simulink library "SimMainLibrary"  (R2017b)
settings: Solver=ode45  StartTime=0.0  StopTime=10.0  RelTol=1e-3  EnableMultiTasking=on
values from neighbouring files (symbols this model uses):
  A = eye(16,16)    [full_input_list.m]
  B = zeros(16,1)    [full_input_list.m]
  C = blkdiag(eye(3,3),zeros(3,3),eye(10,10))    [full_input_list.m]
  centerMass = 2.7719    [full_input_list.m]
  H = C    [full_input_list.m]
  homeClock = clock    [full_input_list.m]    (also in initSimulink.m)
  kane_density = 1000    [full_input_list.m]
  m = 4*1/6    (= 0.666666666667)    [initACS.m]
  mewE = 3.986004418e14    (= 398600441800000)    [full_input_list.m]    (also in initACS.m)
  Q_k = zeros(16,16)    [full_input_list.m]
  R = R_k    [full_input_list.m]
  side1Dim = [ 10 10 6.124 ]/100    [full_input_list.m]
  side1Mass = 0.3283    [full_input_list.m]
  side2Dim = [ 10 10 6.124 ]/100    [full_input_list.m]
  st = 1/freq    (= 0.0125)    [full_input_list.m]    (also in initSimulink.m)
  state1_i = [ 0 0 0 , 0 0 0 , q4_0', w0_N]'    [full_input_list.m]
  state2_i = [ 0 0 (teth_length+side1Dim(1)/2+centerDim(3)/2+10*eps) , 0 -.1 0 ,      q4_0_Cube2' , w0_N ]'    [full_input_list.m]
  state3_i = [ 0 0 -(teth_length+side1Dim(1)/2+centerDim(3)/2+10*eps), 0 .1 0 ,      q4_0_Cube3' , w0_N ]'    [full_input_list.m]
  teth_length = 1    [full_input_list.m]
  teth_numLinks = 3    [full_input_list.m]
  u_k = zeros(16,1)    [full_input_list.m]
  w_k = zeros(16,1)    [full_input_list.m]
  Z_k = zeros(16,1)    [full_input_list.m]
undefined symbols (not defined in the file or in its folder): DiscIntNeverNeededParam, IAU, spring1kd, spring1ks, X, Y, Z
libraries: sm_lib x113, SimMainLibrary x27, nesl_utility x24, simulink x9, sharedutil x2, dspmtrx3 x1, dspinverses x1, aerolibtransform2 x1, aerolibgravity2 x1
(part 7 of 7)

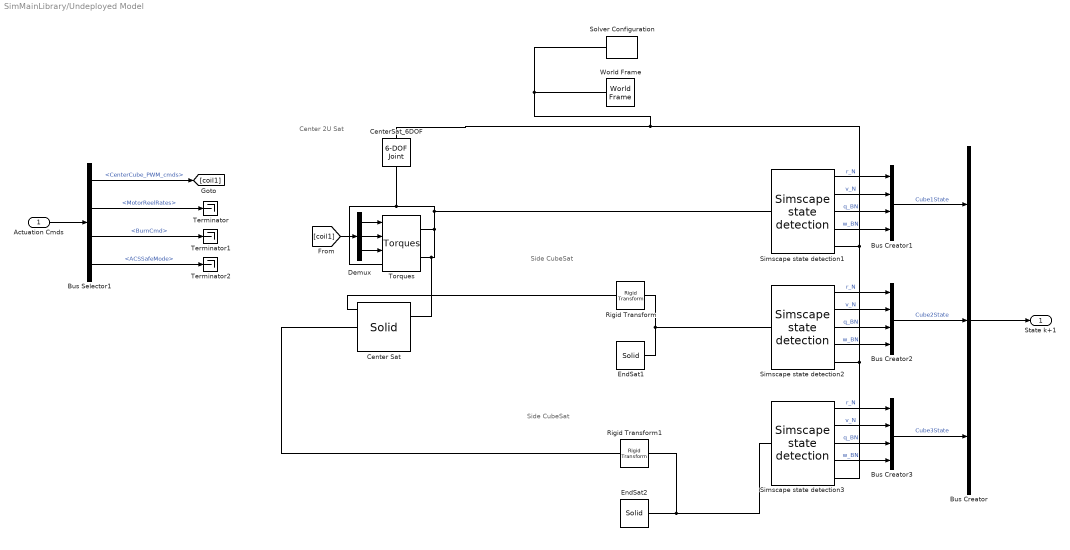
== system SimMainLibrary/Undeployed Model ==
  note: Side CubeSat
  note: Side CubeSat
  note: Center 2U Sat
  Actuation Cmds : Inport
  Bus Creator : BusCreator  Inputs=3
  Bus Creator1 : BusCreator  Inputs=4
  Bus Creator2 : BusCreator  Inputs=4
  Bus Creator3 : BusCreator  Inputs=4
  Bus Selector1 : BusSelector  OutputSignals=CenterCube_PWM_cmds,MotorReelRates,BurnCmd,ACSSafeMode
  Center Sat : sm_lib/Body Elements/Solid  InertiaType=CalculateFromGeometry  Mass=centerMass  MassUnits=kg  CenterOfMass=[0 0 0]  CenterOfMassUnits=m  MomentsOfInertia=[1 1 1]  MomentsOfInertiaUnits=kg*m^2  ProductsOfInertia=[0 0 0]  ProductsOfInertiaUnits=kg*m^2  DensityBased=off  Density=1000  DensityUnits=kg/(m^3)  DoExposeReferenceFrame=on  SerializedFrames=<Frames><Frame><Id>Frame1</Id><Value><Name>PosZ</Name><Origin><Source>GeometricFeature</Source><FeatureName>+z surface</FeatureName></Origin><PrimaryAxis><DefinedDirection>+Z</DefinedDirection><Source>ReferenceFrame</Source><SourceDirection>+Z</SourceDirection><FeatureName></FeatureName></PrimaryAxis><SecondaryAxis><DefinedDirection>+X</DefinedDirection><Source>ReferenceFrame</Source><SourceDirection>+X</SourceDirection><FeatureName></FeatureName></SecondaryAxis></Value></Frame><Frame><Id>Frame2</Id><Value><Name>NegZ</Name><Origin><Source>GeometricFeature</Source><FeatureName>-z surface</FeatureName></Origin><PrimaryAxis><DefinedDirection>+Z</DefinedDirection><Source>ReferenceFrame</Source><SourceDirection>+Z</SourceDirection><FeatureName></FeatureName></PrimaryAxis><SecondaryAxis><DefinedDirection>+X</DefinedDirection><Source>ReferenceFrame</Source><SourceDirection>+X</SourceDirection><FeatureName></FeatureName></SecondaryAxis></Value></Frame><Frame><Id>Frame3</Id><Value><Name>PosY</Name><Origin><Source>ReferenceFrame</Source><FeatureName></FeatureName></Origin><PrimaryAxis><DefinedDirection>+Z</DefinedDirection><Source>ReferenceFrame</Source><SourceDirection>+Z</SourceDirection><FeatureName></FeatureName></PrimaryAxis><SecondaryAxis><DefinedDirection>+X</DefinedDirection><Source>ReferenceFrame</Source><SourceDirection>+X</SourceDirection><FeatureName></FeatureName></SecondaryAxis></Value></Frame><Frame><Id>Frame4</Id><Value><Name>NegY</Name><Origin><Source>ReferenceFrame</Source><FeatureName></FeatureName></Origin><PrimaryAxis><DefinedDirection>+Z</DefinedDirection><Source>ReferenceFrame</Source><SourceDirection>+Z</SourceDirection><FeatureName></FeatureName></PrimaryAxis><SecondaryAxis><DefinedDirection>+X</DefinedDirection><Source>ReferenceFrame</Source><SourceDirection>+X</SourceDirection><FeatureName></FeatureName></SecondaryAxis></Value></Frame></Frames>  GraphicType=FromGeometry  MarkerShape=Sphere  MarkerSize=10  GraphicVisPropType=SimpleVisualProperties  GraphicDiffuseColor=[0.5 0.5 0.5]  GraphicSpecularColor=[0.5 0.5 0.5 1.0]  GraphicAmbientColor=[0.15 0.15 0.15 1.0]  GraphicEmissiveColor=[0.0 0.0 0.0 1.0]  GraphicShininess=75  GraphicOpacity=1.0  GeometryShape=Brick  RectangleSize=[1 1]  RectangleSizeUnits=m  BrickDimensions=centerDim  BrickDimensionUnits=m  CylinderRadius=1  CylinderRadiusUnits=m  CylinderLength=1  CylinderLengthUnits=m  SphereRadius=1  SphereRadiusUnits=m  EllipsoidRadii=[1 1 1]  EllipsoidRadiiUnits=m  ExtrusionCrossSection=[1 1; -1 1; -1 -1; 1 -1]  ExtrusionCrossSectionUnits=m  ExtrusionLength=1  ExtrusionLengthUnits=m  PolygonNumSides=3  PolygonOuterRadius=1  PolygonOuterRadiusUnits=m  ExtGeomFileType=STEP  ExtGeomFileUnits=m  RevolutionCrossSection=[1 1; 1 -1; 2 -1; 2 1]  RevolutionCrossSectionUnits=m  RevolutionExtent=Full  RevolutionAngle=180  RevolutionAngleUnits=deg
  CenterSat_6DOF : sm_lib/Joints/6-DOF Joint  SenseConstraintForce=off  SenseConstraintForceX=off  SenseConstraintForceY=off  SenseConstraintForceZ=off  SenseConstraintTorque=off  SenseConstraintTorqueX=off  SenseConstraintTorqueY=off  SenseConstraintTorqueZ=off  SenseTotalForce=off  SenseTotalForceX=off  SenseTotalForceY=off  SenseTotalForceZ=off  SenseTotalTorque=off  SenseTotalTorqueX=off  SenseTotalTorqueY=off  SenseTotalTorqueZ=off  CompositeWrenchDir=FollowerOnBase  CompositeWrenchFrame=BaseFrame  PxEquilibriumPosition=0  PxEquilibriumPositionUnits=m  PxSpringStiffness=0  PxSpringStiffnessUnits=N/m  PxDampingCoefficient=0  PxDampingCoefficientUnits=N/(m/s)  PxTorqueActuationMode=NoTorque  PxMotionActuationMode=ComputedMotion  PxSensePosition=off  PxSenseVelocity=off  PxSenseAcceleration=off  PxSenseTorqueForce=off  PxPositionTargetSpecify=on  PxPositionTargetPriority=High  PxPositionTargetValue=state1_i(1)  PxPositionTargetValueUnits=m  PxVelocityTargetSpecify=on  PxVelocityTargetPriority=High  PxVelocityTargetValue=state1_i(4)  PxVelocityTargetValueUnits=m/s  PyEquilibriumPosition=0  PyEquilibriumPositionUnits=m  PySpringStiffness=0  PySpringStiffnessUnits=N/m  PyDampingCoefficient=0  PyDampingCoefficientUnits=N/(m/s)  PyTorqueActuationMode=NoTorque  PyMotionActuationMode=ComputedMotion  PySensePosition=off  PySenseVelocity=off  PySenseAcceleration=off  PySenseTorqueForce=off  PyPositionTargetSpecify=on  PyPositionTargetPriority=High  PyPositionTargetValue=state1_i(2)  PyPositionTargetValueUnits=m  PyVelocityTargetSpecify=on  PyVelocityTargetPriority=High  PyVelocityTargetValue=state1_i(5)  PyVelocityTargetValueUnits=m/s  PzEquilibriumPosition=0  PzEquilibriumPositionUnits=m  PzSpringStiffness=0  PzSpringStiffnessUnits=N/m  PzDampingCoefficient=0  PzDampingCoefficientUnits=N/(m/s)  PzTorqueActuationMode=NoTorque  PzMotionActuationMode=ComputedMotion  PzSensePosition=off  PzSenseVelocity=off  PzSenseAcceleration=off  PzSenseTorqueForce=off  PzPositionTargetSpecify=on  PzPositionTargetPriority=High  PzPositionTargetValue=state1_i(3)  PzPositionTargetValueUnits=m  PzVelocityTargetSpecify=on  PzVelocityTargetPriority=High  PzVelocityTargetValue=state1_i(6)  PzVelocityTargetValueUnits=m/s  SphDefPosRotationMethod=None  SphDefPosRotationAngleUnits=deg  SphDefPosRotationStandardAxis=+Z  SphDefPosRotationAngle=0.0  SphDefPosRotationArbitraryAxis=[0 0 1]  SphDefPosFollAlignAxisA=+X  SphDefPosBaseAlignAxisA=+Y  SphDefPosFollAlignAxisB=+Y  SphDefPosBaseAlignAxisB=+Z  SphDefPosRotationSequenceAxes=FollowerAxes  SphDefPosRotationSequence=XYX  SphDefPosRotationSequenceAngles=[0 0 0]  SphDefPosRotationSequenceAnglesUnits=deg  SphDefPosRotationMatrix=[1 0 0; 0 1 0; 0 0 1]  SphEqPosRotationMethod=None  SphEqPosRotationAngleUnits=deg  SphEqPosRotationStandardAxis=+Z  SphEqPosRotationAngle=0.0  SphEqPosRotationArbitraryAxis=[0 0 1]  SphEqPosFollAlignAxisA=+X  SphEqPosBaseAlignAxisA=+Y  SphEqPosFollAlignAxisB=+Y  SphEqPosBaseAlignAxisB=+Z  SphEqPosRotationSequenceAxes=FollowerAxes  SphEqPosRotationSequence=XYX  SphEqPosRotationSequenceAngles=[0 0 0]  SphEqPosRotationSequenceAnglesUnits=deg  SphEqPosRotationMatrix=[1 0 0; 0 1 0; 0 0 1]  SphSpringStiffness=0  SphSpringStiffnessUnits=N*m/deg  SphDampingCoefficient=0  SphDampingCoefficientUnits=N*m/(deg/s)  SphActuateTorqueX=off  SphActuateTorqueY=off  SphActuateTorqueZ=off  SphActuateTorque=off  SphTorqueActuationMode=NoTorque  SphMotionActuationMode=ComputedMotion  SphActuationFrame=BaseFrame  SphSensePosition=off  SphSenseVelocityX=off  SphSenseVelocityY=off  SphSenseVelocityZ=off  SphSenseVelocity=off  SphSenseAccelerationX=off  SphSenseAccelerationY=off  SphSenseAccelerationZ=off  SphSenseAcceleration=off  SphSenseTorqueX=off  SphSenseTorqueY=off  SphSenseTorqueZ=off  SphSenseTorqueForce=off  SphSensingFrame=BaseFrame  SphPositionTargetRotationMethod=RotationMatrix  SphPositionTargetRotationAngleUnits=deg  SphPositionTargetRotationStandardAxis=+Z  SphPositionTargetRotationAngle=0.0  SphPositionTargetRotationArbitraryAxis=[0 0 1]  SphPositionTargetFollAlignAxisA=+X  SphPositionTargetBaseAlignAxisA=+Y  SphPositionTargetFollAlignAxisB=+Y  SphPositionTargetBaseAlignAxisB=+Z  SphPositionTargetRotationSequenceAxes=FollowerAxes  SphPositionTargetRotationSequence=XYX  SphPositionTargetRotationSequenceAngles=[0 0 0]  SphPositionTargetRotationSequenceAnglesUnits=deg  SphPositionTargetRotationMatrix=state1_i_rotation  SphPositionTargetSpecify=on  SphPositionTargetPriority=High  SphVelocityTargetValue=state1_i(11:13)  SphVelocityTargetValueUnits=rad/s  SphVelocityTargetSpecify=on  SphVelocityTargetPriority=High  SphVelocityTargetInFollowerFrame=on
  Demux : Demux  Outputs=3
  EndSat1 : sm_lib/Body Elements/Solid  InertiaType=CalculateFromGeometry  Mass=side1Mass  MassUnits=kg  CenterOfMass=[0 0 0]  CenterOfMassUnits=m  MomentsOfInertia=[1 1 1]  MomentsOfInertiaUnits=kg*m^2  ProductsOfInertia=[0 0 0]  ProductsOfInertiaUnits=kg*m^2  DensityBased=off  Density=1000  DensityUnits=kg/(m^3)  DoExposeReferenceFrame=on  SerializedFrames=<Frames><Frame><Id>Frame1</Id><Value><Name>F1</Name><Origin><Source>GeometricFeature</Source><FeatureName>-y surface</FeatureName></Origin><PrimaryAxis><DefinedDirection>+Z</DefinedDirection><Source>ReferenceFrame</Source><SourceDirection>-Z</SourceDirection><FeatureName></FeatureName></PrimaryAxis><SecondaryAxis><DefinedDirection>+X</DefinedDirection><Source>ReferenceFrame</Source><SourceDirection>+X</SourceDirection><FeatureName></FeatureName></SecondaryAxis></Value></Frame></Frames>  GraphicType=FromGeometry  MarkerShape=Sphere  MarkerSize=10  GraphicVisPropType=SimpleVisualProperties  GraphicDiffuseColor=[0.5 0.5 0.5]  GraphicSpecularColor=[0.5 0.5 0.5 1.0]  GraphicAmbientColor=[0.15 0.15 0.15 1.0]  GraphicEmissiveColor=[0.0 0.0 0.0 1.0]  GraphicShininess=75  GraphicOpacity=1.0  GeometryShape=Brick  RectangleSize=[1 1]  RectangleSizeUnits=m  BrickDimensions=side1Dim  BrickDimensionUnits=m  CylinderRadius=1  CylinderRadiusUnits=m  CylinderLength=1  CylinderLengthUnits=m  SphereRadius=1  SphereRadiusUnits=m  EllipsoidRadii=[1 1 1]  EllipsoidRadiiUnits=m  ExtrusionCrossSection=[1 1; -1 1; -1 -1; 1 -1]  ExtrusionCrossSectionUnits=m  ExtrusionLength=1  ExtrusionLengthUnits=m  PolygonNumSides=3  PolygonOuterRadius=1  PolygonOuterRadiusUnits=m  ExtGeomFileType=STEP  ExtGeomFileUnits=m  RevolutionCrossSection=[1 1; 1 -1; 2 -1; 2 1]  RevolutionCrossSectionUnits=m  RevolutionExtent=Full  RevolutionAngle=180  RevolutionAngleUnits=deg
  EndSat2 : sm_lib/Body Elements/Solid  InertiaType=CalculateFromGeometry  Mass=side1Mass  MassUnits=kg  CenterOfMass=[0 0 0]  CenterOfMassUnits=m  MomentsOfInertia=[1 1 1]  MomentsOfInertiaUnits=kg*m^2  ProductsOfInertia=[0 0 0]  ProductsOfInertiaUnits=kg*m^2  DensityBased=off  Density=1000  DensityUnits=kg/(m^3)  DoExposeReferenceFrame=on  SerializedFrames=<Frames><Frame><Id>Frame1</Id><Value><Name>F1</Name><Origin><Source>GeometricFeature</Source><FeatureName>-y surface</FeatureName></Origin><PrimaryAxis><DefinedDirection>+Z</DefinedDirection><Source>ReferenceFrame</Source><SourceDirection>-Z</SourceDirection><FeatureName></FeatureName></PrimaryAxis><SecondaryAxis><DefinedDirection>+X</DefinedDirection><Source>ReferenceFrame</Source><SourceDirection>+X</SourceDirection><FeatureName></FeatureName></SecondaryAxis></Value></Frame></Frames>  GraphicType=FromGeometry  MarkerShape=Sphere  MarkerSize=10  GraphicVisPropType=SimpleVisualProperties  GraphicDiffuseColor=[0.5 0.5 0.5]  GraphicSpecularColor=[0.5 0.5 0.5 1.0]  GraphicAmbientColor=[0.15 0.15 0.15 1.0]  GraphicEmissiveColor=[0.0 0.0 0.0 1.0]  GraphicShininess=75  GraphicOpacity=1.0  GeometryShape=Brick  RectangleSize=[1 1]  RectangleSizeUnits=m  BrickDimensions=side1Dim  BrickDimensionUnits=m  CylinderRadius=1  CylinderRadiusUnits=m  CylinderLength=1  CylinderLengthUnits=m  SphereRadius=1  SphereRadiusUnits=m  EllipsoidRadii=[1 1 1]  EllipsoidRadiiUnits=m  ExtrusionCrossSection=[1 1; -1 1; -1 -1; 1 -1]  ExtrusionCrossSectionUnits=m  ExtrusionLength=1  ExtrusionLengthUnits=m  PolygonNumSides=3  PolygonOuterRadius=1  PolygonOuterRadiusUnits=m  ExtGeomFileType=STEP  ExtGeomFileUnits=m  RevolutionCrossSection=[1 1; 1 -1; 2 -1; 2 1]  RevolutionCrossSectionUnits=m  RevolutionExtent=Full  RevolutionAngle=180  RevolutionAngleUnits=deg
  Rigid Transform : sm_lib/Frames and Transforms/Rigid Transform  TranslationMethod=Cartesian  TranslationStandardOffset=0  TranslationLengthUnit=m  TranslationStandardAxis=+Z  TranslationCartesianOffset=[0 0 side1Dim(3)/2]  TranslationROffset=0  TranslationROffsetUnits=m  TranslationZOffset=0  TranslationZOffsetUnits=m  TranslationThetaOffset=0  TranslationThetaOffsetUnits=deg  RotationMethod=None  RotationAngleUnits=deg  RotationStandardAxis=+Z  RotationAngle=0.0  RotationArbitraryAxis=[0 0 1]  FollAlignAxisA=+X  BaseAlignAxisA=+Y  FollAlignAxisB=+Y  BaseAlignAxisB=+Z  RotationSequenceAxes=FollowerAxes  RotationSequence=XYX  RotationSequenceAngles=[0 0 0]  RotationSequenceAnglesUnits=deg  RotationMatrix=[1 0 0; 0 1 0; 0 0 1]
  Rigid Transform1 : sm_lib/Frames and Transforms/Rigid Transform  TranslationMethod=Cartesian  TranslationStandardOffset=0  TranslationLengthUnit=m  TranslationStandardAxis=+Z  TranslationCartesianOffset=[0 0 -side2Dim(3)/2]  TranslationROffset=0  TranslationROffsetUnits=m  TranslationZOffset=0  TranslationZOffsetUnits=m  TranslationThetaOffset=0  TranslationThetaOffsetUnits=deg  RotationMethod=None  RotationAngleUnits=deg  RotationStandardAxis=+Z  RotationAngle=0.0  RotationArbitraryAxis=[0 0 1]  FollAlignAxisA=+X  BaseAlignAxisA=+Y  FollAlignAxisB=+Y  BaseAlignAxisB=+Z  RotationSequenceAxes=FollowerAxes  RotationSequence=XYX  RotationSequenceAngles=[0 0 0]  RotationSequenceAnglesUnits=deg  RotationMatrix=[1 0 0; 0 1 0; 0 0 1]
  Simscape state detection1 : SimMainLibrary/Simscape state detection
      settings: SourceProductName=CUGravity Library
  Simscape state detection2 : SimMainLibrary/Simscape state detection
      settings: SourceProductName=CUGravity Library
  Simscape state detection3 : SimMainLibrary/Simscape state detection
      settings: SourceProductName=CUGravity Library
  Solver Configuration : nesl_utility/Solver Configuration  PhysicalDomain=network_engine_domain  SubClassName=solver  LeftPortType=input  RightPortType=generic  Accelerate=off  Tones=[]  Harmonics=[]  SimulateNoise=off  Profile=off  UseLocalSampling=off  EnableSwitchedLinearOptims=on  FrequencyDomain=off  UseCCode=off  RelTol=0.001  AbsTol=1e-06  MinStep=1e-09  ToWorkspace=off  RevertToSquareIcSolve=off  NumHomotopyIterations=100  PhasorMode=off  PhasorModeNumHarmonics=1  DoDC=off  ResidualTolerance=1e-09  UseLocalSolver=off  LocalSolverChoice=NE_BACKWARD_EULER_ADVANCER  LocalSolverSampleTime=st  DoFixedCost=off  MaxNonlinIter=3  MaxModeIter=2  LinearAlgebra=Sparse  DelaysMemoryBudget=1024  AutomaticFiltering=off  FilteringTimeConstant=0.001
  Terminator : Terminator
  Terminator1 : Terminator
  Terminator2 : Terminator
  Torques : SimMainLibrary/Single Link Simscape Model/Torques
      settings: SourceProductName=CUGravity Library
  World Frame : sm_lib/Frames and Transforms/World Frame
  State k+1 : Outport
  wires:
  Actuation Cmds/1 -> Bus Selector1/1
  Simscape state detection3/4 -> Bus Creator3/4  "w_BN"
  Simscape state detection3/3 -> Bus Creator3/3  "q_BN"
  Simscape state detection3/2 -> Bus Creator3/2  "v_N"
  Simscape state detection3/1 -> Bus Creator3/1  "r_N"
  Simscape state detection2/4 -> Bus Creator2/4  "w_BN"
  Simscape state detection2/3 -> Bus Creator2/3  "q_BN"
  Simscape state detection2/2 -> Bus Creator2/2  "v_N"
  Simscape state detection2/1 -> Bus Creator2/1  "r_N"
  Simscape state detection1/4 -> Bus Creator1/4  "w_BN"
  Simscape state detection1/3 -> Bus Creator1/3  "q_BN"
  Simscape state detection1/2 -> Bus Creator1/2  "v_N"
  Simscape state detection1/1 -> Bus Creator1/1  "r_N"
  Bus Creator3/1 -> Bus Creator/3  "Cube3State"
  Bus Creator2/1 -> Bus Creator/2  "Cube2State"
  Bus Creator1/1 -> Bus Creator/1  "Cube1State"
  Bus Creator/1 -> State k+1/1
  Demux/2 -> Torques/2
  Demux/3 -> Torques/3
  Demux/1 -> Torques/1
  [coil1] -> Demux/1
  Bus Selector1/1 -> [coil1]  "<CenterCube_PWM_cmds>"
  Bus Selector1/2 -> Terminator/1  "<MotorReelRates>"
  Bus Selector1/3 -> Terminator1/1  "<BurnCmd>"
  Bus Selector1/4 -> Terminator2/1  "<ACSSafeMode>"
  connections:
  Torques/RConn2 -- Center Sat/RConn1 -- Torques/RConn1 -- CenterSat_6DOF/RConn1 -- Torques/LConn1 -- Simscape state detection1/LConn1
  Solver Configuration/RConn1 -- Simscape state detection3/RConn1 -- Simscape state detection2/RConn1 -- Simscape state detection1/RConn1 -- CenterSat_6DOF/LConn1 -- World Frame/RConn1
  EndSat1/RConn1 -- Rigid Transform/RConn1 -- Simscape state detection2/LConn1
  EndSat2/RConn1 -- Rigid Transform1/RConn1 -- Simscape state detection3/LConn1
  Rigid Transform/LConn1 -- Center Sat/LConn1
  Rigid Transform1/LConn1 -- Center Sat/LConn2

== system SimMainLibrary/Update Tether properties ==
  note: Update Tether properties
  note: Update Tether Properties
      | This block updates the dynamic properties of the tether in response to input from MotorReelRates.
      | It outputs a continuous signal of the current tether length for use in the SimScape models.
      | If there is a non-zero reeling signal, it updates the dynamic variables in the workspace.
  <MotorReelRates> : Inport
  Abs : Abs
  Add : Sum
  Add1 : Sum
  Add2 : Sum
  Constant1 : Constant  Value=teth_length
  Constant4 : Constant  Value=teth_length
  If : If  IfExpression=u1 > 1e-5  ShowElse=off
  If Action Subsystem : Subsystem  TreatAsAtomicUnit=on
  Length Signal Filter : TransferFcn  Denominator=[.02 .25 1]
  Mux : Mux  Inputs=3
  Terminator : Terminator  Commented=on
  Unit Delay : UnitDelay  SampleTime=-1
  Tether length : Outport
  Out1 : Outport  Port=2
  wires:
  If/1 -> If Action Subsystem/Action
  <MotorReelRates>/1 -> Mux/1, Add/2, If Action Subsystem/1(Length Increment), Abs/1  "Controller Signal"
  Constant4/1 -> Add1/1
  Add/1 -> Length Signal Filter/1, Add1/2, Mux/2, Unit Delay/1  "Added Length"
  Add1/1 -> If Action Subsystem/2(Length)  "Length"
  Unit Delay/1 -> Add/1
  Abs/1 -> If/1
  Mux/1 -> Out1/1
  Add2/1 -> Tether length/1, Mux/3
  Length Signal Filter/1 -> Add2/1
  Constant1/1 -> Add2/2

== system SimMainLibrary/cross product matrix ==
  a : Inport
  Constant : Constant  Value=0
  Constant1 : Constant  Value=0
  Constant7 : Constant  Value=0
  Demux : Demux  Outputs=3
  Gain2 : Gain  Gain=-1
  Gain3 : Gain  Gain=-1
  Gain4 : Gain  Gain=-1
  crs : sharedutil/Create 3x3 Matrix
  ax : Outport
  wires:
  crs/1 -> ax/1
  Constant/1 -> crs/1
  Constant1/1 -> crs/5
  Constant7/1 -> crs/9
  Gain2/1 -> crs/2
  Demux/1 -> crs/8, Gain3/1
  Demux/2 -> crs/3, Gain4/1
  Gain4/1 -> crs/7
  a/1 -> Demux/1
  Demux/3 -> crs/4, Gain2/1
  Gain3/1 -> crs/6

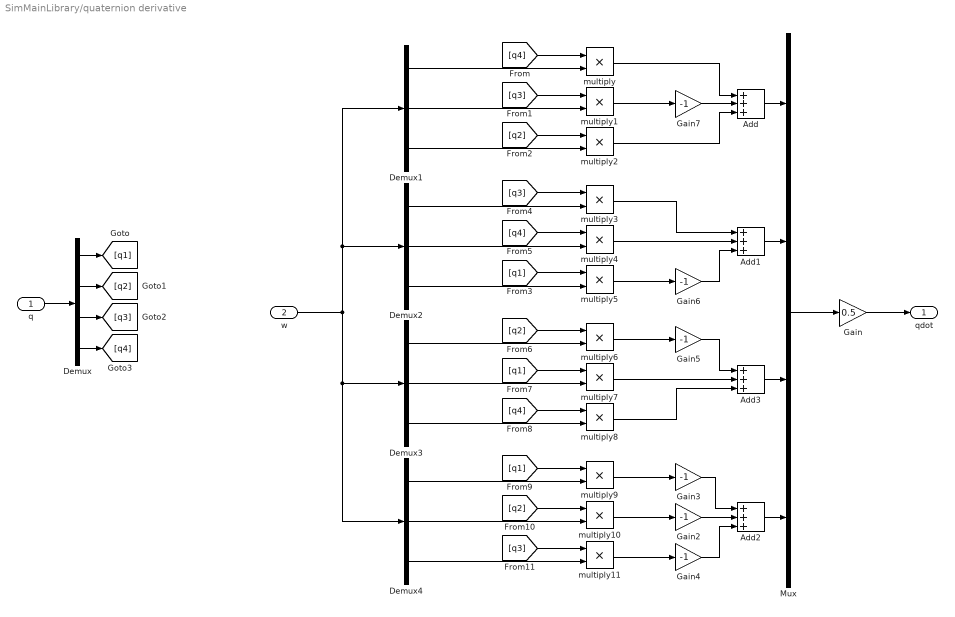
== system SimMainLibrary/quaternion derivative ==
  q : Inport
  w : Inport  Port=2
  Add{,1..3} (4 alike) : Sum  Inputs=+++
  Demux : Demux
  Demux{1..4} (4 alike) : Demux  Outputs=3
  Gain : Gain  Gain=0.5
  Gain{2..7} (6 alike) : Gain  Gain=-1
  Mux : Mux
  multiply{,1..11} (12 alike) : Product  Inputs=**
  qdot : Outport
  wires:
  Add/1 -> Mux/1
  Gain2/1 -> Add2/2
  Gain6/1 -> Add1/3
  Add3/1 -> Mux/3
  Add2/1 -> Mux/4
  Add1/1 -> Mux/2
  multiply/1 -> Add/1
  multiply1/1 -> Gain7/1
  Gain4/1 -> Add2/3
  Gain3/1 -> Add2/1
  Gain7/1 -> Add/2
  Mux/1 -> Gain/1
  multiply4/1 -> Add1/2
  multiply5/1 -> Gain6/1
  Gain5/1 -> Add3/1
  multiply7/1 -> Add3/2
  multiply10/1 -> Gain2/1
  multiply8/1 -> Add3/3
  multiply3/1 -> Add1/1
  multiply2/1 -> Add/3
  multiply9/1 -> Gain3/1
  multiply11/1 -> Gain4/1
  multiply6/1 -> Gain5/1
  q/1 -> Demux/1
  w/1 -> Demux3/1, Demux4/1, Demux2/1, Demux1/1
  Gain/1 -> qdot/1
  Demux1/2 -> multiply1/2
  Demux1/1 -> multiply/2
  Demux1/3 -> multiply2/2
  Demux2/1 -> multiply3/2
  Demux2/2 -> multiply4/2
  Demux2/3 -> multiply5/2
  Demux3/1 -> multiply6/2
  Demux3/2 -> multiply7/2
  Demux3/3 -> multiply8/2
  Demux4/3 -> multiply11/2
  Demux4/2 -> multiply10/2
  Demux4/1 -> multiply9/2
  Demux/1 -> [q1]
  Demux/2 -> [q2]
  Demux/3 -> [q3]
  Demux/4 -> [q4]
  [q4] -> multiply/1
  [q3] -> multiply1/1
  [q2] -> multiply2/1
  [q1] -> multiply5/1
  [q3] -> multiply3/1
  [q4] -> multiply4/1
  [q2] -> multiply6/1
  [q1] -> multiply7/1
  [q4] -> multiply8/1
  [q1] -> multiply9/1
  [q2] -> multiply10/1
  [q3] -> multiply11/1

== system SimMainLibrary/Sequential Motor Controller/Spinning fast1 ==
  In1 : Inport
  Action Port : ActionPort  InitializeStates=reset
  Out1 : Outport
  wires:
  In1/1 -> Out1/1

== system SimMainLibrary/Sequential Motor Controller/Spinning slow1 ==
  Action Port : ActionPort
  Constant : Constant  Value=0
  Out1 : Outport
  wires:
  Constant/1 -> Out1/1

== system SimMainLibrary/SideCubeEstimators/Kalman Gain and Estamated State Computation ==
  P_kp : Inport
  x_kp : Inport  Port=2
  Y : Inport  Port=3
  " LU Inverse" : dspinverses/ LU Inverse
      settings: SourceProductName=DSP System Toolbox
  Add1 : Sum
  Add3 : Sum  Inputs=-+
  H : Constant  Value=H
  H1 : Constant  Value=H
  Math Function : Math  Operator=transpose  SaturateOnIntegerOverflow=on
  Product{,1,3..4,6} (5 alike) : Product  Multiplication=Matrix(*)
  R : Constant  Value=R
  K : Outport
  x_k : Outport  Port=2
  wires:
  Add3/1 -> x_k/1
  P_kp/1 -> Product1/1, Product3/2
  Product6/1 -> Add3/1
  H1/1 -> Product6/1
  Product3/1 -> Product4/1
  Add1/1 -> " LU Inverse"/1
  Product4/1 -> Add1/1
  R/1 -> Add1/2
  Y/1 -> Add3/2
  x_kp/1 -> Product6/2
  Product/1 -> K/1  "Kalman Gain K"
  Math Function/1 -> Product4/2
  Product1/1 -> Product/1
  " LU Inverse"/1 -> Product/2
  H/1 -> Math Function/1, Product1/2, Product3/1

== system SimMainLibrary/SideCubeEstimators/New State Prediction  ==
  P_k-1 : Inport
  x_k-1 : Inport  Port=2
  A : Constant  Value=A
  Add1 : Sum  Inputs=+++
  Add2 : Sum
  B : Constant  Value=B
  Math Function : Math  Operator=transpose  SaturateOnIntegerOverflow=on
  Product{,1..3} (4 alike) : Product  Multiplication=Matrix(*)
  Q_k : Constant  Value=Q_k
  u_k : Constant  Value=u_k
  w_k : Constant  Value=w_k
  P_kp : Outport
  "x_kp  " : Outport  Port=2
  wires:
  Add2/1 -> P_kp/1
  Product3/1 -> Add2/1
  P_k-1/1 -> Product2/2
  Q_k/1 -> Add2/2
  Add1/1 -> "x_kp  "/1
  w_k/1 -> Add1/3
  u_k/1 -> Product1/2
  Product1/1 -> Add1/2
  B/1 -> Product1/1
  A/1 -> Product/1, Product2/1, Math Function/1
  x_k-1/1 -> Product/2
  Product/1 -> Add1/1
  Math Function/1 -> Product3/2
  Product2/1 -> Product3/1

== system SimMainLibrary/SideCubeEstimators/Y computation ==
  In1 : Inport
  Add2 : Sum
  C : Constant  Value=C
  Product2 : Product  Multiplication=Matrix(*)
  "Z_k " : Constant  Value=Z_k
  Y : Outport
  wires:
  Product2/1 -> Add2/1
  C/1 -> Product2/1
  In1/1 -> Product2/2
  "Z_k "/1 -> Add2/2
  Add2/1 -> Y/1

== system SimMainLibrary/SideCubeSensors/Create Mag Vector ==
  q_BN : Inport
  r_N : Inport  Port=2
  Constant : Constant  Value=[1 1 1]
  Terminator : Terminator
  Terminator1 : Terminator
  mag_B : Outport
  wires:
  q_BN/1 -> Terminator/1
  r_N/1 -> Terminator1/1
  Constant/1 -> mag_B/1

== system SimMainLibrary/SideCubeSensors/Create Sun Vector ==
  q_BN : Inport
  r_N : Inport  Port=2
  time : Inport  Port=3
  Constant1 : Constant  Value=[1 1 1]
  Terminator : Terminator
  Terminator1 : Terminator
  Terminator2 : Terminator
  sun_B : Outport
  wires:
  q_BN/1 -> Terminator/1
  r_N/1 -> Terminator1/1
  Constant1/1 -> sun_B/1
  time/1 -> Terminator2/1

== system SimMainLibrary/SideCubeSensors/Frame Convert ==
  a_N : Inport
  q_BN : Inport  Port=2
  Terminator : Terminator
  a_B : Outport
  wires:
  a_N/1 -> a_B/1
  q_BN/1 -> Terminator/1

== system SimMainLibrary/Single Link Simscape Model/Torques ==
  tau_Y : Inport
  tau_X : Inport  Port=2
  tau_Z : Inport  Port=3
  External Force and Torque : sm_lib/Forces and Torques/External Force and Torque  ForceResolutionFrame=AttachedFrame  EnableForceX=off  EnableForceY=off  EnableForceZ=off  EnableForce=off  TorqueResolutionFrame=AttachedFrame  EnableTorqueX=off  EnableTorqueY=on  EnableTorqueZ=off  EnableTorque=off
  External Force and Torque1 : sm_lib/Forces and Torques/External Force and Torque  ForceResolutionFrame=AttachedFrame  EnableForceX=off  EnableForceY=off  EnableForceZ=off  EnableForce=off  TorqueResolutionFrame=AttachedFrame  EnableTorqueX=on  EnableTorqueY=off  EnableTorqueZ=off  EnableTorque=off
  External Force and Torque2 : sm_lib/Forces and Torques/External Force and Torque  ForceResolutionFrame=AttachedFrame  EnableForceX=off  EnableForceY=off  EnableForceZ=off  EnableForce=off  TorqueResolutionFrame=AttachedFrame  EnableTorqueX=off  EnableTorqueY=off  EnableTorqueZ=on  EnableTorque=off
  Simulink-PS Converter : nesl_utility/Simulink-PS Converter  PhysicalDomain=network_engine_domain  SubClassName=ps_input  LeftPortType=input  RightPortType=output  PseudoPeriodic=off  Frequencies=[]  NoiseDistribution=none  NoiseParameters=[]  Unit=1  AffineConversion=off  FilteringAndDerivatives=zero  SimscapeFilterOrder=1  InputFilterTimeConstant=0.001  UdotUserProvided=1
  Simulink-PS Converter1 : nesl_utility/Simulink-PS Converter  PhysicalDomain=network_engine_domain  SubClassName=ps_input  LeftPortType=input  RightPortType=output  PseudoPeriodic=off  Frequencies=[]  NoiseDistribution=none  NoiseParameters=[]  Unit=1  AffineConversion=off  FilteringAndDerivatives=zero  SimscapeFilterOrder=1  InputFilterTimeConstant=0.001  UdotUserProvided=1
  Simulink-PS Converter2 : nesl_utility/Simulink-PS Converter  PhysicalDomain=network_engine_domain  SubClassName=ps_input  LeftPortType=input  RightPortType=output  PseudoPeriodic=off  Frequencies=[]  NoiseDistribution=none  NoiseParameters=[]  Unit=1  AffineConversion=off  FilteringAndDerivatives=zero  SimscapeFilterOrder=1  InputFilterTimeConstant=0.001  UdotUserProvided=1
  torY : PMIOPort  Port=1  Side=Right
  torX : PMIOPort  Port=2  Side=Right
  torZ : PMIOPort  Port=3  Side=Left
  wires:
  tau_Z/1 -> Simulink-PS Converter2/1
  tau_X/1 -> Simulink-PS Converter1/1
  tau_Y/1 -> Simulink-PS Converter/1
  connections:
  External Force and Torque2/LConn1 -- Simulink-PS Converter2/RConn1
  External Force and Torque2/RConn1 -- torZ/RConn1
  External Force and Torque1/LConn1 -- Simulink-PS Converter1/RConn1
  External Force and Torque/LConn1 -- Simulink-PS Converter/RConn1
  External Force and Torque1/RConn1 -- torX/RConn1
  External Force and Torque/RConn1 -- torY/RConn1

== system SimMainLibrary/Update Tether properties/If Action Subsystem ==
  Length Increment : Inport
  Length : Inport  Port=2
  Action Port : ActionPort
  Constant : Constant  Value=teth_numLinks
  Constant2 : Constant  Value=spring1ks
  Constant3 : Constant  Value=spring1kd
  Demux : Demux  Commented=on  Outputs=3
  Interpreted MATLAB Function : MATLABFcn  MATLABFcn=updateTetherProps  OutputDimensions=0  Output1D=off
  Mux : Mux  Inputs=5
  Terminator : Terminator
  Terminator1 : Terminator
  Terminator2 : Terminator
  Terminator3 : Terminator  Commented=on
  wires:
  Demux/3 -> Terminator2/1
  Demux/2 -> Terminator1/1
  Demux/1 -> Terminator/1
  Mux/1 -> Interpreted MATLAB Function/1
  Length/1 -> Mux/2
  Constant3/1 -> Mux/5
  Constant2/1 -> Mux/4
  Length Increment/1 -> Mux/3
  Constant/1 -> Mux/1
